simulink model "MathACM601"  (R2018b)
settings: Solver=FixedStepAuto  StartTime=0.0  StopTime=Tmu*100  FixedStep=Ts1  RelTol=1e-3
values from neighbouring files (symbols this model uses):
  add_error = 0    [MathACM601.m]
  ce = 0.0712    [MathACM601.m]
  cm = 0.0712    [MathACM601.m]
  comp = 0    [MathACM601.m]
  delU = 0    [MathACM601.m]
  dia = 0.002*Isc*kdt    (= 13.339872)    [MathACM601.m]
  dib = 0.003*Isc*kdt    (= 20.009808)    [MathACM601.m]
  dic = -0.009*Isc*kdt    (= -60.029424)    [MathACM601.m]
  Ibias = Ubias/Rshunt/Kopa    (= 3.09182195233)    [MathACM601.m]
  J = 0.11e-4    (= 1.1e-05)    [MathACM601.m]
  k = 2    [MathACM601.m]
  KADC = (2^12-1)/3.3    (= 1240.90909091)    [MathACM601.m]
  kda = 1    [MathACM601.m]
  kdb = 0.99    [MathACM601.m]
  kdc = 1.015    [MathACM601.m]
  kdt = Rshunt*Kopa*KADC    (= 625.3065)    [MathACM601.m]
  Ki1 = 1/(Kob*Tt)    (= 375)    [MathACM601.m]
  Ki2 = J*2/(3*8*Tmu^2*ce)    (= 0.514981273408)    [MathACM601.m]
  Kopa = 1.527    [MathACM601.m]
  Kp1 = Te*Ki1    (= 0.5625)    [MathACM601.m]
  Kp2 = 4*Tmu*Ki2    (= 0.0102996254682)    [MathACM601.m]
  Kv = 1    [MathACM601.m]
  Lsa = Ls    (= 0.002)    [MathACM601.m]
  Lsb = Ls    (= 0.002)    [MathACM601.m]
  Lsc = Ls    (= 0.002)    [MathACM601.m]
  Mm1 = 2.232    [MathACM601.m]
  Mm2 = 0.565    [MathACM601.m]
  Nc = 72    [MathACM601.m]
  Q1 = -90.7*pi/180    (= -1.58301363156)    [MathACM601.m]
  Q2 = -61*pi/180    (= -1.06465084372)    [MathACM601.m]
  R = 0.75    [MathACM601.m]
  Ra = R    (= 0.75)    [MathACM601.m]
  Rb = R    (= 0.75)    [MathACM601.m]
  Rc = R    (= 0.75)    [MathACM601.m]
  Rshunt = 0.33    [MathACM601.m]
  Sw = 0    [MathACM601.m]
  tau = 0.00    (= 0)    [MathACM601.m]
  Te = R*Ls    (= 0.0015)    [MathACM601.m]
  Tmu = 10*Tt    (= 0.005)    [MathACM601.m]
  Ts1 = 0.5e-4    (= 5e-05)    [MathACM601.m]
  Ts2 = 0.5e-3    (= 0.0005)    [MathACM601.m]
  Tt = Ts1*10    (= 0.0005)    [MathACM601.m]
  turn_M = 0    [MathACM601.m]
  Tz = Ts1/2    (= 2.5e-05)    [MathACM601.m]
  Ubias = 1.558    [MathACM601.m]
  Udc = 8    [MathACM601.m]
  zp = 4    [MathACM601.m]
settings Model: Creator=ivshu  LastModifiedBy=Шустов Илья
settings SFSimCC: SimUseLocalCustomCode=off
settings RTWCC: RTWUseLocalCustomCode=off
settings CodeAppCC: StateflowObjectComments=on
settings SimscapeCC: SimscapeNormalizeSystem=off

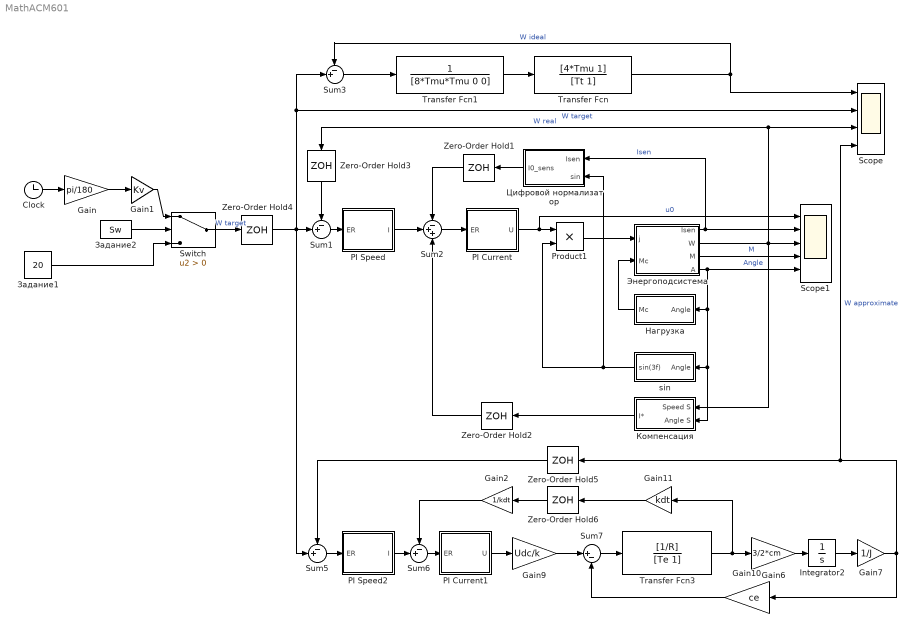
== system MathACM601 ==
  Clock : Clock
  Gain : Gain  Gain=pi/180
  Gain1 : Gain  Gain=Kv
  Gain10 : Gain  Gain=ce
  Gain11 : Gain  Gain=kdt
  Gain2 : Gain  Gain=1/kdt
  Gain6 : Gain  Gain=3/2*cm
  Gain7 : Gain  Gain=1/J
  Gain9 : Gain  Gain=Udc/k
  Integrator2 : Integrator
  PI Current : Subsystem
  PI Current1 : Subsystem
  PI Speed : Subsystem
  PI Speed2 : Subsystem
  Product1 : Product
  Scope : Scope  NumInputPorts=4
  Scope1 : Scope  NumInputPorts=5
  Sum{1,3,5..6} (4 alike) : Sum  Inputs=-+|
  Sum2 : Sum  Inputs=-++
  Sum7 : Sum  Inputs=|+-
  Switch : Switch  Criteria=u2 > Threshold
  Transfer Fcn : TransferFcn  Numerator=[4*Tmu 1]  Denominator=[Tt 1]
  Transfer Fcn1 : TransferFcn  Denominator=[8*Tmu*Tmu 0 0]
  Transfer Fcn3 : TransferFcn  Numerator=[1/R]  Denominator=[Te 1]
  Zero-Order Hold1 : ZeroOrderHold  SampleTime=Ts1
  Zero-Order Hold2 : ZeroOrderHold  SampleTime=Ts1
  Zero-Order Hold3 : ZeroOrderHold  SampleTime=Ts2
  Zero-Order Hold4 : ZeroOrderHold  SampleTime=Ts2
  Zero-Order Hold5 : ZeroOrderHold  SampleTime=Ts2
  Zero-Order Hold6 : ZeroOrderHold  SampleTime=Ts1
  sin : Subsystem
  Задание1 : Constant  Value=20
  Задание2 : Constant  Value=Sw
  Компенсация : Subsystem
  Нагрузка : Subsystem
  Цифровой нормализатор : Subsystem
  Энергоподсистема : Subsystem
  wires:
  sin/1(sin(3f)) -> Product1/2, Цифровой нормализатор/2(sin)
  Product1/1 -> Энергоподсистема/1(j)
  Энергоподсистема/2(W) -> Компенсация/1(Speed S), Scope1/3, Zero-Order Hold3/1, Scope/3  "W real"
  Sum2/1 -> PI Current/1(ER)
  Zero-Order Hold1/1 -> Sum2/1
  Zero-Order Hold3/1 -> Sum1/1
  Задание1/1 -> Switch/3
  Gain/1 -> Gain1/1
  Clock/1 -> Gain/1
  Gain1/1 -> Switch/1
  Энергоподсистема/4(A) -> Компенсация/2(Angle S), sin/1(Angle), Нагрузка/1(Angle), Scope1/5  "Angle"
  Нагрузка/1(Mc) -> Энергоподсистема/2(Mc)
  Энергоподсистема/1(Isen) -> Цифровой нормализатор/1(Isen), Scope1/2  "Isen"
  Switch/1 -> Zero-Order Hold4/1  "W target"
  Задание2/1 -> Switch/2
  Компенсация/1(I*) -> Zero-Order Hold2/1
  Zero-Order Hold2/1 -> Sum2/3
  Transfer Fcn1/1 -> Transfer Fcn/1
  Transfer Fcn/1 -> Sum3/1, Scope/1  "W ideal"
  Sum1/1 -> PI Speed/1(ER)
  Sum5/1 -> PI Speed2/1(ER)
  PI Speed2/1(I) -> Sum6/2
  Sum6/1 -> PI Current1/1(ER)
  PI Current1/1(U) -> Gain9/1
  Transfer Fcn3/1 -> Gain6/1, Gain11/1
  Integrator2/1 -> Gain7/1
  Gain6/1 -> Integrator2/1
  Gain7/1 -> Gain10/1, Scope/4, Zero-Order Hold5/1  "W approximate"
  Zero-Order Hold5/1 -> Sum5/1
  Zero-Order Hold6/1 -> Gain2/1
  Sum7/1 -> Transfer Fcn3/1
  Gain9/1 -> Sum7/1
  Gain10/1 -> Sum7/2
  Gain11/1 -> Zero-Order Hold6/1
  Sum3/1 -> Transfer Fcn1/1
  PI Current/1(U) -> Scope1/1, Product1/1  "u0"
  PI Speed/1(I) -> Sum2/2
  Цифровой нормализатор/1(I0_sens) -> Zero-Order Hold1/1
  Энергоподсистема/3(M) -> Scope1/4  "M"
  Gain2/1 -> Sum6/1
  Zero-Order Hold4/1 -> Sum5/2, Sum3/2, Scope/2, Sum1/2  "W target"

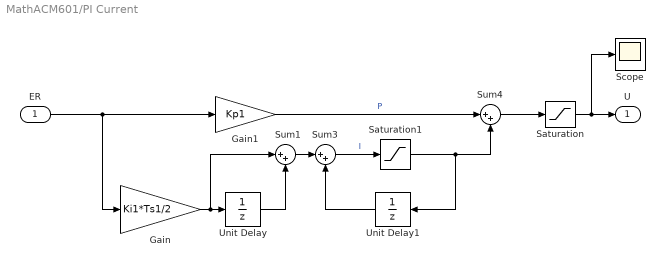
== system MathACM601/PI Current ==
  ER : Inport
  Gain : Gain  Gain=Ki1*Ts1/2
  Gain1 : Gain  Gain=Kp1
  Saturation : Saturate  UpperLimit=1  LowerLimit=-1
  Saturation1 : Saturate  UpperLimit=1  LowerLimit=-1
  Scope : Scope
  Sum1 : Sum  Inputs=|++
  Sum3 : Sum  Inputs=|++
  Sum4 : Sum  Inputs=|++
  Unit Delay : UnitDelay  SampleTime=Ts1
  Unit Delay1 : UnitDelay  SampleTime=Ts1
  U : Outport
  wires:
  Saturation/1 -> Scope/1, U/1
  Sum4/1 -> Saturation/1
  Gain/1 -> Sum1/1, Unit Delay/1
  Unit Delay/1 -> Sum1/2
  Sum1/1 -> Sum3/1
  Unit Delay1/1 -> Sum3/2
  Sum3/1 -> Saturation1/1  "I"
  Gain1/1 -> Sum4/1  "P"
  ER/1 -> Gain/1, Gain1/1
  Saturation1/1 -> Sum4/2, Unit Delay1/1

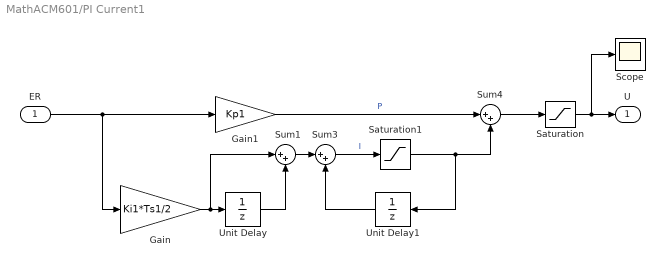
== system MathACM601/PI Current1 ==
  ER : Inport
  Gain : Gain  Gain=Ki1*Ts1/2
  Gain1 : Gain  Gain=Kp1
  Saturation : Saturate  UpperLimit=1  LowerLimit=-1
  Saturation1 : Saturate  UpperLimit=1  LowerLimit=-1
  Scope : Scope
  Sum1 : Sum  Inputs=|++
  Sum3 : Sum  Inputs=|++
  Sum4 : Sum  Inputs=|++
  Unit Delay : UnitDelay  SampleTime=Ts1
  Unit Delay1 : UnitDelay  SampleTime=Ts1
  U : Outport
  wires:
  Saturation/1 -> Scope/1, U/1
  Sum4/1 -> Saturation/1
  Gain/1 -> Sum1/1, Unit Delay/1
  Unit Delay/1 -> Sum1/2
  Sum1/1 -> Sum3/1
  Unit Delay1/1 -> Sum3/2
  Sum3/1 -> Saturation1/1  "I"
  Gain1/1 -> Sum4/1  "P"
  ER/1 -> Gain/1, Gain1/1
  Saturation1/1 -> Sum4/2, Unit Delay1/1

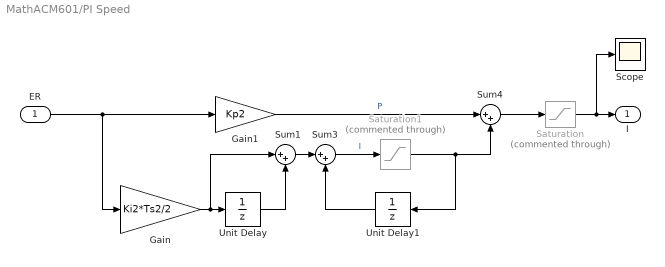
== system MathACM601/PI Speed ==
  ER : Inport
  Gain : Gain  Gain=Ki2*Ts2/2
  Gain1 : Gain  Gain=Kp2
  Saturation : Saturate  Commented=through  UpperLimit=1  LowerLimit=-1
  Saturation1 : Saturate  Commented=through  UpperLimit=1  LowerLimit=-1
  Scope : Scope
  Sum1 : Sum  Inputs=|++
  Sum3 : Sum  Inputs=|++
  Sum4 : Sum  Inputs=|++
  Unit Delay : UnitDelay  SampleTime=Ts2
  Unit Delay1 : UnitDelay  SampleTime=Ts2
  I : Outport
  wires:
  Sum4/1 -> Saturation/1
  Gain/1 -> Sum1/1, Unit Delay/1
  Unit Delay/1 -> Sum1/2
  Sum1/1 -> Sum3/1
  Unit Delay1/1 -> Sum3/2
  Sum3/1 -> Saturation1/1  "I"
  Gain1/1 -> Sum4/1  "P"
  ER/1 -> Gain/1, Gain1/1
  Saturation1/1 -> Sum4/2, Unit Delay1/1
  Saturation/1 -> Scope/1, I/1

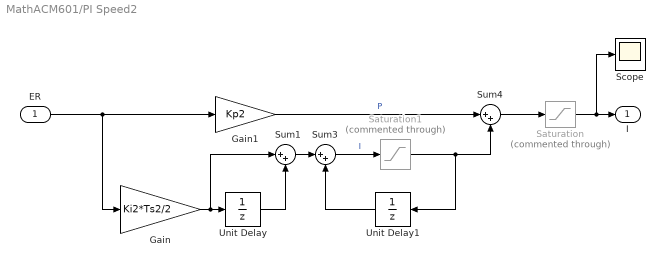
== system MathACM601/PI Speed2 ==
  ER : Inport
  Gain : Gain  Gain=Ki2*Ts2/2
  Gain1 : Gain  Gain=Kp2
  Saturation : Saturate  Commented=through  UpperLimit=1  LowerLimit=-1
  Saturation1 : Saturate  Commented=through  UpperLimit=1  LowerLimit=-1
  Scope : Scope
  Sum1 : Sum  Inputs=|++
  Sum3 : Sum  Inputs=|++
  Sum4 : Sum  Inputs=|++
  Unit Delay : UnitDelay  SampleTime=Ts2
  Unit Delay1 : UnitDelay  SampleTime=Ts2
  I : Outport
  wires:
  Sum4/1 -> Saturation/1
  Gain/1 -> Sum1/1, Unit Delay/1
  Unit Delay/1 -> Sum1/2
  Sum1/1 -> Sum3/1
  Unit Delay1/1 -> Sum3/2
  Sum3/1 -> Saturation1/1  "I"
  Gain1/1 -> Sum4/1  "P"
  ER/1 -> Gain/1, Gain1/1
  Saturation1/1 -> Sum4/2, Unit Delay1/1
  Saturation/1 -> Scope/1, I/1

== system MathACM601/sin ==
  Angle : Inport
  Fcn1 : Fcn  Expr=sin(u(1))
  Fcn2 : Fcn  Expr=sin(u(1)+2*pi/3)
  Fcn3 : Fcn  Expr=sin(u(1)-2*pi/3)
  Gain2 : Gain  Gain=zp
  Mux2 : Mux  Inputs=3
  sin(3f) : Outport
  wires:
  Fcn2/1 -> Mux2/2
  Fcn3/1 -> Mux2/3
  Fcn1/1 -> Mux2/1
  Mux2/1 -> sin(3f)/1
  Angle/1 -> Gain2/1
  Gain2/1 -> Fcn1/1, Fcn3/1, Fcn2/1

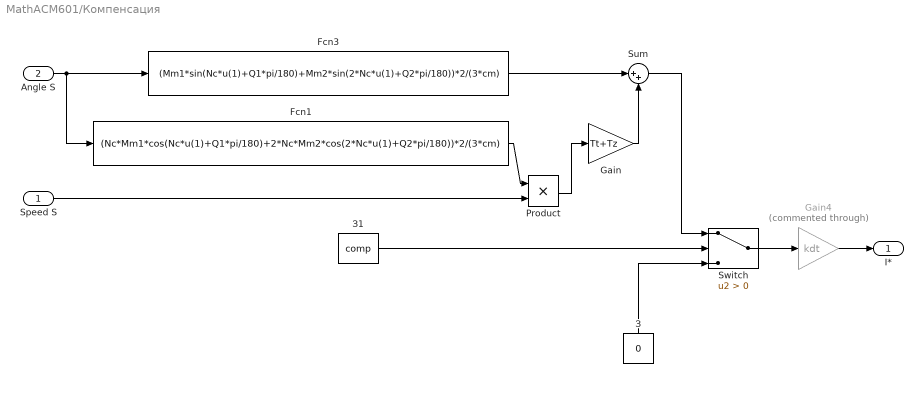
== system MathACM601/Компенсация ==
  Speed S : Inport
  Angle S : Inport  Port=2
  Fcn1 : Fcn  Expr=(Nc*Mm1*cos(Nc*u(1)+Q1*pi/180)+2*Nc*Mm2*cos(2*Nc*u(1)+Q2*pi/180))*2/(3*cm)
  Fcn3 : Fcn  Expr=(Mm1*sin(Nc*u(1)+Q1*pi/180)+Mm2*sin(2*Nc*u(1)+Q2*pi/180))*2/(3*cm)
  Gain : Gain  Gain=Tt+Tz
  Gain4 : Gain  Commented=through  Gain=kdt
  Product : Product
  Sum : Sum  Inputs=|++
  Switch : Switch  Criteria=u2 > Threshold
  З : Constant  Value=0
  З1 : Constant  Value=comp
  I* : Outport
  wires:
  Angle S/1 -> Fcn3/1, Fcn1/1
  Sum/1 -> Switch/1
  З/1 -> Switch/3
  З1/1 -> Switch/2
  Switch/1 -> Gain4/1
  Fcn3/1 -> Sum/1
  Speed S/1 -> Product/2
  Fcn1/1 -> Product/1
  Product/1 -> Gain/1
  Gain/1 -> Sum/2
  Gain4/1 -> I*/1

== system MathACM601/Нагрузка ==
  Angle : Inport
  Fcn1 : Fcn  Expr=Mm1*sin(Nc*u(1)+Q1*pi/180)+Mm2*sin(Nc*2*u(1)+Q2*pi/180)
  Switch : Switch  Criteria=u2 > Threshold
  З : Constant  Value=0.01
  Переключатель : Constant  Value=turn_M
  Mc : Outport
  wires:
  Switch/1 -> Mc/1
  Fcn1/1 -> Switch/1
  З/1 -> Switch/3
  Angle/1 -> Fcn1/1
  Переключатель/1 -> Switch/2

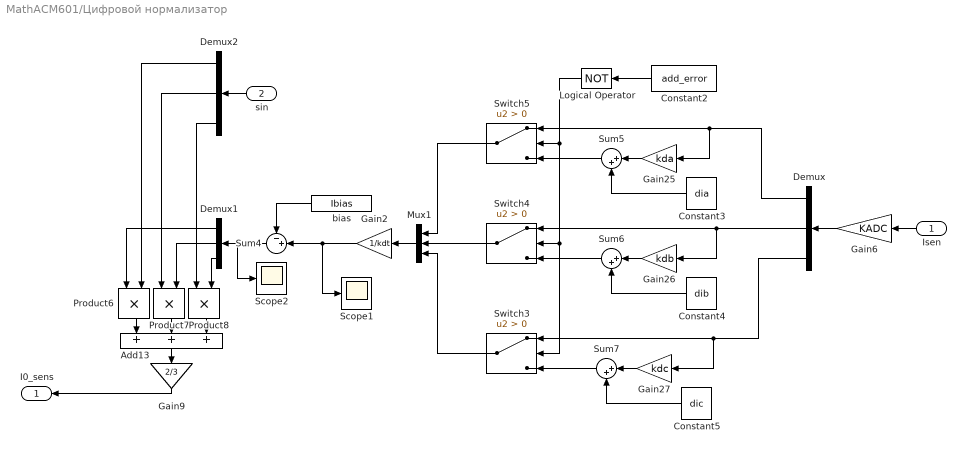
== system MathACM601/Цифровой нормализатор ==
  Isen : Inport
  sin : Inport  Port=2
  Add13 : Sum  Inputs=+++
  Constant2 : Constant  Value=add_error
  Constant3 : Constant  Value=dia
  Constant4 : Constant  Value=dib
  Constant5 : Constant  Value=dic
  Demux : Demux  Outputs=3
  Demux1 : Demux  Outputs=3
  Demux2 : Demux  Outputs=3
  Gain2 : Gain  Gain=1/kdt
  Gain25 : Gain  Gain=kda
  Gain26 : Gain  Gain=kdb
  Gain27 : Gain  Gain=kdc
  Gain6 : Gain  Gain=KADC
  Gain9 : Gain  Gain=2/3
  Logical Operator : Logic  Operator=NOT  AllPortsSameDT=off  OutDataTypeStr=boolean
  Mux1 : Mux  Inputs=3
  Product6 : Product
  Product7 : Product
  Product8 : Product
  Scope1 : Scope
  Scope2 : Scope
  Sum4 : Sum  Inputs=-+|
  Sum5 : Sum  Inputs=|++
  Sum6 : Sum  Inputs=|++
  Sum7 : Sum  Inputs=|++
  Switch3 : Switch  Criteria=u2 > Threshold
  Switch4 : Switch  Criteria=u2 > Threshold
  Switch5 : Switch  Criteria=u2 > Threshold
  bias : Constant  Value=Ibias
  I0_sens : Outport
  wires:
  Switch4/1 -> Mux1/2
  Switch3/1 -> Mux1/3
  Switch5/1 -> Mux1/1
  Sum5/1 -> Switch5/3
  Constant2/1 -> Logical Operator/1
  Constant3/1 -> Sum5/2
  Gain25/1 -> Sum5/1
  Gain26/1 -> Sum6/1
  Isen/1 -> Gain6/1
  Sum6/1 -> Switch4/3
  Gain27/1 -> Sum7/1
  Sum7/1 -> Switch3/3
  Constant4/1 -> Sum6/2
  Constant5/1 -> Sum7/2
  Logical Operator/1 -> Switch4/2, Switch3/2, Switch5/2
  Demux/3 -> Gain27/1, Switch3/1
  Demux/2 -> Gain26/1, Switch4/1
  Demux/1 -> Gain25/1, Switch5/1
  Sum4/1 -> Scope2/1, Demux1/1
  Demux2/3 -> Product8/1
  Demux2/1 -> Product6/2
  Demux1/2 -> Product7/2
  Product6/1 -> Add13/1
  Product7/1 -> Add13/2
  Demux1/1 -> Product6/1
  Product8/1 -> Add13/3
  Gain9/1 -> I0_sens/1
  Add13/1 -> Gain9/1
  Demux1/3 -> Product8/2
  Mux1/1 -> Gain2/1
  Demux2/2 -> Product7/1
  sin/1 -> Demux2/1
  Gain6/1 -> Demux/1
  Gain2/1 -> Scope1/1, Sum4/2
  bias/1 -> Sum4/1

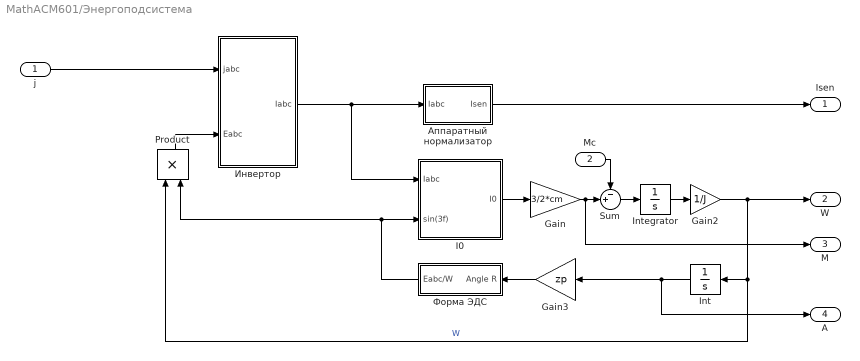
== system MathACM601/Энергоподсистема ==
  j : Inport
  Mc : Inport  Port=2
  Gain : Gain  Gain=3/2*cm
  Gain2 : Gain  Gain=1/J
  Gain3 : Gain  Gain=zp
  I0 : Subsystem
  Int : Integrator
  Integrator : Integrator
  Product : Product
  Sum : Sum  Inputs=-+|
  Аппаратный нормализатор : Subsystem
  Инвертор : Subsystem
  Форма ЭДС : Subsystem
  Isen : Outport
  W : Outport  Port=2
  M : Outport  Port=3
  A : Outport  Port=4
  wires:
  Integrator/1 -> Gain2/1
  j/1 -> Инвертор/1(" jabc")
  Gain2/1 -> Product/1, Int/1, W/1  "W"
  I0/1(I0) -> Gain/1
  Форма ЭДС/1(Eabc/W) -> Product/2, I0/2(sin(3f))
  Sum/1 -> Integrator/1
  Gain3/1 -> Форма ЭДС/1(Angle R)
  Product/1 -> Инвертор/2(Eabc)
  Gain/1 -> M/1, Sum/2
  Инвертор/1(Iabc) -> Аппаратный нормализатор/1(Iabc), I0/1(Iabc)
  Mc/1 -> Sum/1
  Аппаратный нормализатор/1(Isen) -> Isen/1
  Int/1 -> A/1, Gain3/1

== system MathACM601/Энергоподсистема/I0 ==
  Iabc : Inport
  sin(3f) : Inport  Port=2
  Add1 : Sum  Inputs=+++
  Demux1 : Demux  Outputs=3
  Demux2 : Demux  Outputs=3
  Gain1 : Gain  Gain=2/3
  Product1 : Product
  Product2 : Product
  Product3 : Product
  I0 : Outport
  wires:
  sin(3f)/1 -> Demux1/1
  Demux1/3 -> Product3/1
  Demux1/2 -> Product2/1
  Demux1/1 -> Product1/2
  Product3/1 -> Add1/3
  Demux2/1 -> Product1/1
  Add1/1 -> Gain1/1
  Demux2/3 -> Product3/2
  Iabc/1 -> Demux2/1
  Product1/1 -> Add1/1
  Product2/1 -> Add1/2
  Demux2/2 -> Product2/2
  Gain1/1 -> I0/1

== system MathACM601/Энергоподсистема/Аппаратный нормализатор ==
  Iabc : Inport
  Constant1 : Constant  Value=Ubias
  Gain1 : Gain  Gain=Rshunt
  Gain30 : Gain  Gain=Kopa
  Sum1 : Sum  Inputs=++|
  Isen : Outport
  wires:
  Gain1/1 -> Gain30/1
  Constant1/1 -> Sum1/1
  Gain30/1 -> Sum1/2
  Iabc/1 -> Gain1/1
  Sum1/1 -> Isen/1

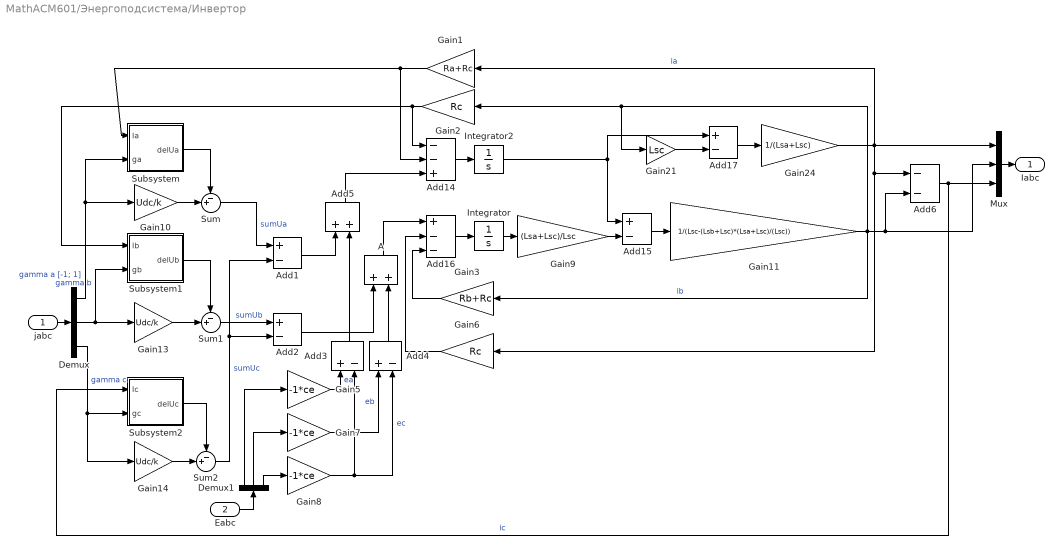
== system MathACM601/Энергоподсистема/Инвертор ==
  " jabc" : Inport
  Eabc : Inport  Port=2
  A : Sum
  Add{1..4,15,17} (6 alike) : Sum  Inputs=+-
  Add14 : Sum  Inputs=--+
  Add16 : Sum  Inputs=+--
  Add5 : Sum
  Add6 : Sum  Inputs=--
  Demux : Demux  Outputs=3
  Demux1 : Demux  Outputs=3
  Gain1 : Gain  Gain=Ra+Rc
  Gain10 : Gain  Gain=Udc/k
  Gain11 : Gain  Gain=1/(Lsc-(Lsb+Lsc)*(Lsa+Lsc)/(Lsc))
  Gain13 : Gain  Gain=Udc/k
  Gain14 : Gain  Gain=Udc/k
  Gain2 : Gain  Gain=Rc
  Gain21 : Gain  Gain=Lsc
  Gain24 : Gain  Gain=1/(Lsa+Lsc)
  Gain3 : Gain  Gain=Rb+Rc
  Gain5 : Gain  Gain=-1*ce
  Gain6 : Gain  Gain=Rc
  Gain7 : Gain  Gain=-1*ce
  Gain8 : Gain  Gain=-1*ce
  Gain9 : Gain  Gain=(Lsa+Lsc)/Lsc
  Integrator : Integrator
  Integrator2 : Integrator
  Mux : Mux  Inputs=3
  Subsystem : Subsystem
  Subsystem1 : Subsystem
  Subsystem2 : Subsystem
  Sum : Sum  Inputs=-+|
  Sum1 : Sum  Inputs=-+|
  Sum2 : Sum  Inputs=-+|
  Iabc : Outport
  wires:
  Demux1/2 -> Gain7/1
  Demux1/3 -> Gain8/1
  Demux1/1 -> Gain5/1
  Demux/1 -> Subsystem/2(ga), Gain10/1  "gamma a [-1; 1]"
  Add6/1 -> Subsystem2/1(Ic), Mux/3  "ic"
  Demux/2 -> Subsystem1/2(gb), Gain13/1  "gamma b"
  Demux/3 -> Subsystem2/2(gc), Gain14/1  "gamma c"
  Add1/1 -> Add5/1
  Gain24/1 -> Mux/1, Gain1/1, Gain6/1, Add6/1  "ia"
  Add14/1 -> Integrator2/1
  Gain1/1 -> Add14/2, Subsystem/1(Ia)
  Integrator/1 -> Gain9/1
  Subsystem1/1(delUb) -> Sum1/1
  A/1 -> Add16/1
  Subsystem/1(delUa) -> Sum/1
  Gain7/1 -> Add4/1  "eb"
  Gain5/1 -> Add3/1  "ea"
  Sum1/1 -> Add2/1  "sumUb"
  Add2/1 -> A/1
  Sum2/1 -> Add2/2, Add1/2  "sumUc"
  Add5/1 -> Add14/3
  Gain2/1 -> Add14/1, Subsystem1/1(Ib)
  Add4/1 -> A/2
  Add16/1 -> Integrator/1
  Gain11/1 -> Gain3/1, Mux/2, Add6/2, Gain21/1, Gain2/1  "ib"
  Gain8/1 -> Add4/2, Add3/2  "ec"
  Sum/1 -> Add1/1  "sumUa"
  Add3/1 -> Add5/2
  Gain21/1 -> Add17/2
  Gain3/1 -> Add16/3
  Gain9/1 -> Add15/2
  Add15/1 -> Gain11/1
  Integrator2/1 -> Add17/1, Add15/1
  Gain6/1 -> Add16/2
  Add17/1 -> Gain24/1
  Gain14/1 -> Sum2/2
  Gain13/1 -> Sum1/2
  Gain10/1 -> Sum/2
  Subsystem2/1(delUc) -> Sum2/1
  " jabc"/1 -> Demux/1
  Eabc/1 -> Demux1/1
  Mux/1 -> Iabc/1

== system MathACM601/Энергоподсистема/Форма ЭДС ==
  Angle R : Inport
  Fcn1 : Fcn  Expr=sin(u(1))
  Fcn2 : Fcn  Expr=sin(u(1)+2*pi/3)
  Fcn3 : Fcn  Expr=sin(u(1)-2*pi/3)
  Mux2 : Mux  Inputs=3
  Eabc/W : Outport
  wires:
  Fcn2/1 -> Mux2/2
  Fcn3/1 -> Mux2/3
  Fcn1/1 -> Mux2/1
  Mux2/1 -> Eabc/W/1
  Angle R/1 -> Fcn2/1, Fcn1/1, Fcn3/1

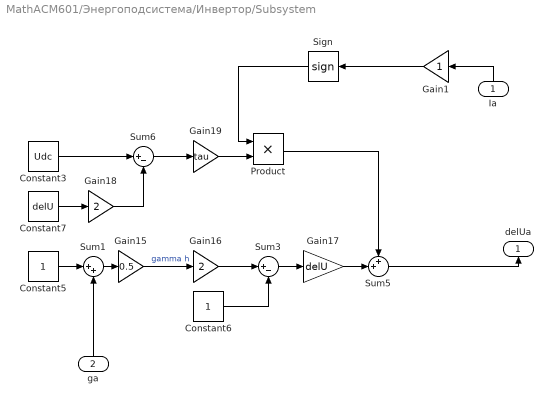
== system MathACM601/Энергоподсистема/Инвертор/Subsystem ==
  Ia : Inport
  ga : Inport  Port=2
  Constant3 : Constant  Value=Udc
  Constant5 : Constant
  Constant6 : Constant
  Constant7 : Constant  Value=delU
  Gain1 : Gain
  Gain15 : Gain  Gain=0.5
  Gain16 : Gain  Gain=2
  Gain17 : Gain  Gain=delU
  Gain18 : Gain  Gain=2
  Gain19 : Gain  Gain=tau
  Product : Product
  Sign : Signum
  Sum1 : Sum  Inputs=|++
  Sum3 : Sum  Inputs=|+-
  Sum5 : Sum  Inputs=++|
  Sum6 : Sum  Inputs=|+-
  delUa : Outport
  wires:
  Sum1/1 -> Gain15/1
  Sum6/1 -> Gain19/1
  Gain16/1 -> Sum3/1
  Product/1 -> Sum5/1
  Sign/1 -> Product/1
  Sum3/1 -> Gain17/1
  Constant6/1 -> Sum3/2
  Constant5/1 -> Sum1/1
  Gain15/1 -> Gain16/1  "gamma h"
  Sum5/1 -> delUa/1
  Gain19/1 -> Product/2
  Ia/1 -> Gain1/1
  ga/1 -> Sum1/2
  Constant3/1 -> Sum6/1
  Gain17/1 -> Sum5/2
  Constant7/1 -> Gain18/1
  Gain18/1 -> Sum6/2
  Gain1/1 -> Sign/1

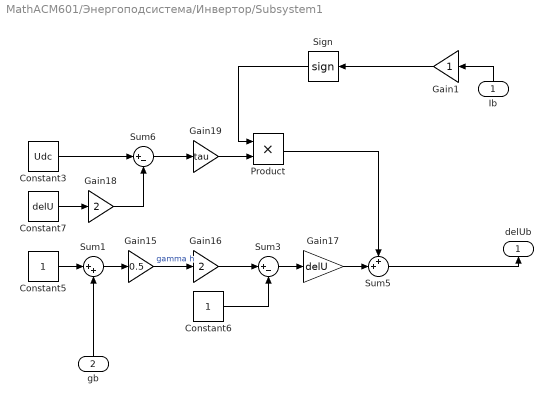
== system MathACM601/Энергоподсистема/Инвертор/Subsystem1 ==
  Ib : Inport
  gb : Inport  Port=2
  Constant3 : Constant  Value=Udc
  Constant5 : Constant
  Constant6 : Constant
  Constant7 : Constant  Value=delU
  Gain1 : Gain
  Gain15 : Gain  Gain=0.5
  Gain16 : Gain  Gain=2
  Gain17 : Gain  Gain=delU
  Gain18 : Gain  Gain=2
  Gain19 : Gain  Gain=tau
  Product : Product
  Sign : Signum
  Sum1 : Sum  Inputs=|++
  Sum3 : Sum  Inputs=|+-
  Sum5 : Sum  Inputs=++|
  Sum6 : Sum  Inputs=|+-
  delUb : Outport
  wires:
  Sum1/1 -> Gain15/1
  Sum6/1 -> Gain19/1
  Gain16/1 -> Sum3/1
  Product/1 -> Sum5/1
  Sign/1 -> Product/1
  Sum3/1 -> Gain17/1
  Constant6/1 -> Sum3/2
  Constant5/1 -> Sum1/1
  Gain15/1 -> Gain16/1  "gamma h"
  Sum5/1 -> delUb/1
  Gain19/1 -> Product/2
  Ib/1 -> Gain1/1
  gb/1 -> Sum1/2
  Constant3/1 -> Sum6/1
  Gain17/1 -> Sum5/2
  Constant7/1 -> Gain18/1
  Gain18/1 -> Sum6/2
  Gain1/1 -> Sign/1

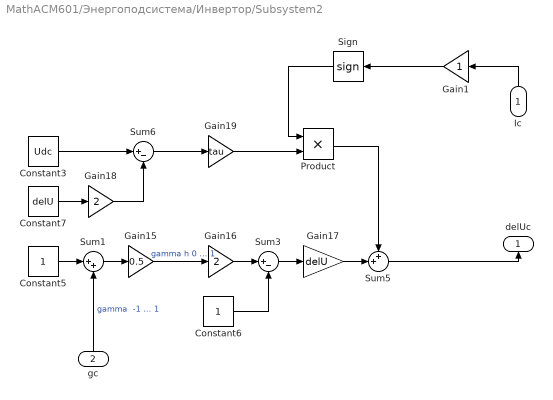
== system MathACM601/Энергоподсистема/Инвертор/Subsystem2 ==
  Ic : Inport
  gc : Inport  Port=2
  Constant3 : Constant  Value=Udc
  Constant5 : Constant
  Constant6 : Constant
  Constant7 : Constant  Value=delU
  Gain1 : Gain
  Gain15 : Gain  Gain=0.5
  Gain16 : Gain  Gain=2
  Gain17 : Gain  Gain=delU
  Gain18 : Gain  Gain=2
  Gain19 : Gain  Gain=tau
  Product : Product
  Sign : Signum
  Sum1 : Sum  Inputs=|++
  Sum3 : Sum  Inputs=|+-
  Sum5 : Sum  Inputs=++|
  Sum6 : Sum  Inputs=|+-
  delUc : Outport
  wires:
  Sum1/1 -> Gain15/1
  Sum6/1 -> Gain19/1
  Gain16/1 -> Sum3/1
  Product/1 -> Sum5/1
  Sign/1 -> Product/1
  Sum3/1 -> Gain17/1
  Constant6/1 -> Sum3/2
  Constant5/1 -> Sum1/1
  Gain15/1 -> Gain16/1  "gamma h 0 ... 1"
  Sum5/1 -> delUc/1
  Gain19/1 -> Product/2
  Ic/1 -> Gain1/1
  gc/1 -> Sum1/2  "gamma  -1 ... 1"
  Constant3/1 -> Sum6/1
  Gain17/1 -> Sum5/2
  Constant7/1 -> Gain18/1
  Gain18/1 -> Sum6/2
  Gain1/1 -> Sign/1
